simulink model "filter_test"  (R2018a)
settings: Solver=VariableStepAuto  StartTime=0.0  StopTime=10  RelTol=1e-3
libraries: dsparch4 x2, simulink x1, dspxfrm3 x1
settings Model: Creator=Na-Teng  LastModifiedBy=Na-Teng

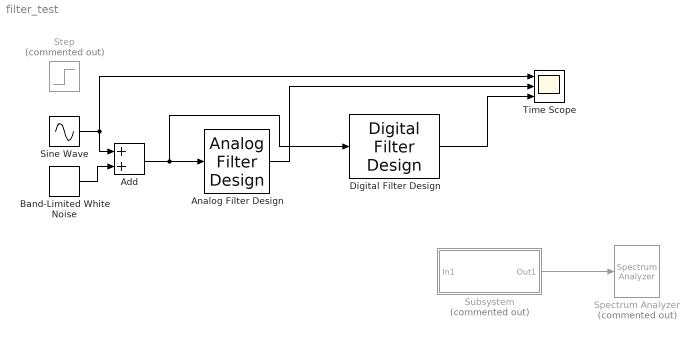
== system filter_test ==
  Add : Sum
  Analog Filter Design : dsparch4/Analog Filter Design  method=Butterworth  filttype=Bandpass  N=8  Wlo=0.1  Whi=5  Rp=2  Rs=40
  Band-Limited White Noise : simulink/Sources/Band-Limited White Noise  Cov=[0.1]  Ts=0.1  seed=[23341]
  Digital Filter Design : dsparch4/Digital Filter Design  mwdsp_browser_bugfix_var=off
  Sine Wave : Sin  Frequency=1000  SampleTime=0
  Spectrum Analyzer : SpectrumAnalyzer  Commented=on
  Step : Step  Commented=on  SampleTime=0
  Subsystem : Subsystem  Commented=on
  Time Scope : Scope  NumInputPorts=3
  wires:
  Subsystem/1(Out1) -> Spectrum Analyzer/1
  Sine Wave/1 -> Time Scope/1, Add/1
  Band-Limited White Noise/1 -> Add/2
  Add/1 -> Digital Filter Design/1, Analog Filter Design/1
  Analog Filter Design/1 -> Time Scope/2
  Digital Filter Design/1 -> Time Scope/3

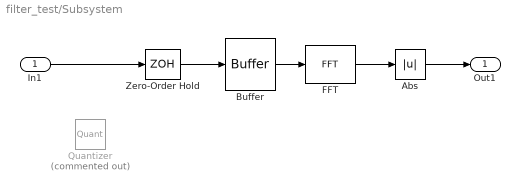
== system filter_test/Subsystem ==
  In1 : Inport
  Abs : Abs
  Buffer : Buffer  N=1536  OutputFrames=off
  FFT : dspxfrm3/FFT  FFTImplementation=Auto  CompMethod=Table lookup  TableOpt=NEW  TableOptActive=Speed  BitRevOrder=off  Normalize=off  InheritFFTLength=on  FFTLength=64  WrapInput=on  roundingMode=Floor  overflowMode=off  firstCoeffDataTypeStr=Inherit: Same word length as input  firstCoeffLastDataTypeStr=Inherit: Same word length as input  outputMin=[]  outputMax=[]
  Quantizer : Quantizer  Commented=on
  Zero-Order Hold : ZeroOrderHold  SampleTime=-1
  Out1 : Outport
  wires:
  Zero-Order Hold/1 -> Buffer/1
  Buffer/1 -> FFT/1
  FFT/1 -> Abs/1
  Abs/1 -> Out1/1
  In1/1 -> Zero-Order Hold/1
